simulink model "MySystem"  (Simulink 4.00)
settings: Solver=ode5  SolverMode=SingleTasking  StartTime=0.0  StopTime=999999  FixedStep=0.01  RelTol=1e-3  AbsTol=1e-6
undefined symbols (not defined in the file): ABSPositionScale, ABSPowerScale, ABSTemperatureScale, ABSVelocityScale, mex_baseaddress
libraries: simulink_extras x2
settings Model: Creator=jims  LastModifiedBy=Administrator  ExternalInput=[]  SaveTime=off  SaveOutput=off  InitialState=[]  LimitDataPoints=off  MaxDataPoints=5000  IntegerOverflowMsg=none  SimulationMode=external  RTWSystemTargetFile=rtwin.tlc  RTWOptions="-aCCOptimize=1 -aEnforceIntegerDowncast=1 -aExtMode=1 -aFoldNonRolledExpr=1 -aForceParamTrailComments=0 -aGenerateComments=1 -aGenerateReport=0 -aIncDataTypeInIds=0 -aIncHierarchyInIds=0 -aInlineInvariantSignals=0 -aInlineParameters=0 -aInlinedPrmAccess=\"Literals\" -aLocalBlockOutputs=1 -aMaxRTWIdLen=31 -aPrefixModelToSubsysFcnNames=1 -aRTWVerbose=1 -aRebuildAll=0 -aRollThreshold=5 -aShowEliminatedStatements=1"  RTWTemplateMakefile=abs_win_vc.tmf  ExtModeMexFile=rtwinext  ExtModeTrigDuration=6000  BlockReductionOpt=off

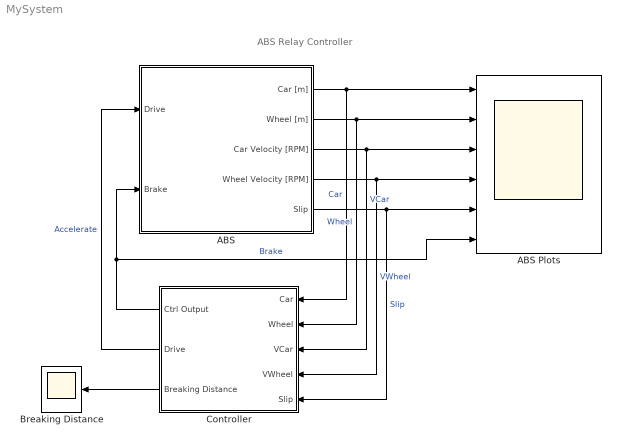
== system MySystem ==
  note: ABS Relay Controller
  ABS : Subsystem  mask{BaseAddress=mex_baseaddress(-1,-1), T0=0.01}
      mask prompts: BaseAddress "Base Address"; T0 "Sample Time"
      settings: RTWFcnNameOpts=Auto  RTWFileNameOpts=Auto
      mask Display: plot([-0.2 -0.2], [-0.2 -0.2], [1.2 1.2], [1.2 1.2], [0.9 0.9], [0.6 0.9], [0.9 0.9], [0.3 0.5], [0.85 0.85 0.95 0.95], [0.7 0.5 0.5 0.7], [0.75 0.75], [0.8 0.9], [0.75 0.75], [0.3 0.4], [0.75 0.775], [0.4 0.425], [0.775 0.725 0.775], [0.425 0.475 0.525], [0.775 0.725 0.775], [0.525 0.575 0.625], [0.775 0.725 0.775], [0.625 0.675 0.725], [0.775 0.725 0.75], [0.725 0.775 0.8], [0.65 0.95], [0.9 0.9], [0.65 0.7], [0.9 1], [0.7 0.75], [0.9 1], [0.75 0.8], [0.9 1], [0.8 0.85], [0.9 1], [0.85 0.9], [0.9 1], [0.9 0.95], [0.9 1], [0.95 1], [0.9 1], 0.4+0.3*sin([0 0.20 0.41 0.62 0.83 1.04 1.25 1.46 1.67 1.88 2.09 2.30 2.51 2.72 2.93 3.14 3.35 3.56 3.76 3.97 4.18 4.39 4.60 4.81 5.02 5.23 5.44 5.65 5.86 6.07 6.28]), 0.3+0.3*cos([0 0.20 0.41 0.62 0.83 1.04 1.25 1.46 1.67 1.88 2.09 2.30 2.51 2.72 2.93 3.14 3.35 3.56 3.76 3.97 4.18 4.39 4.60 4.81 5.02 5.23 5.44 5.65 5.86 6.07 6.28]), (1-0.005)+0.005*sin([0 0.20 0.41 0.62 0.83 1.04 1.25 1.46 1.67 1.88 2.09 2.30 2.51 2.72 2.93 3.14 3.35 3.56 3.76 3.97 4.18 4.39 4.60 4.81 5.02 5.23 5.44 5.65 5.86 6.07 6.28]), 0.3+0.005*cos([0 0.20 0.41 0.62 0.83 1.04 1.25 1.46 1.67 1.88 2.09 2.30 2.51 2.72 2.93 3.14 3.35 3.56 3.76 3.97 4.18 4.39 4.60 4.81 5.02 5.23 5.44 5.65 5.86 6.07 6.28]), 0.4+0.005*sin([0 0.20 0.41 0.62 0.83 1.04 1.25 1.46 1.67 1.88 2.09 2.30 2.51 2.72 2.93 3.14 3.35 3.56 3.76 3.97 4.18 4.39 4.60 4.81 5.02 5.23 5.44 5.65 5.86 6.07 6.28]), 0.3+0.005*cos([0 0.20 0.41 0.62 0.83 1.04 1.25 1.46 1.67 1.88 2.09 2.30 2.51 2.72 2.93 3.14 3.35 3.56 3.76 3.97 4.18 4.39 4.60 4.81 5.02 5.23 5.44 5.65 5.86 6.07 6.28]), [0.4 1], [0.3 0.3], [0 1], [0 0] )
  ABS Plots : Scope  NumInputPorts=6
      settings: TimeRange=30  YMin=0~0~0~0~-0.05~0  YMax=140~140~1750~1750~0.3~1  SaveName=ABSHistory  LimitDataPoints=on  MaxDataPoints=6000
  Breaking Distance : Scope
      settings: TimeRange=30  YMin=0  YMax=15  SaveName=ABSBreakingWay  LimitDataPoints=on  MaxDataPoints=6000
  Controller : Subsystem  Orientation=left  mask(ABS Relay Controller){VelTr=1700, SwPoint=[0.1 0.1], CntLevel=[0 1]}
      mask prompts: VelTr "Velocity Treshold [RPM]:"; SwPoint "Switch Point [ON OFF]:"; CntLevel "Control When [ON OFF]:"
      mask help: Parameters of the ABS relay controller
      settings: RTWFcnNameOpts=Auto  RTWFileNameOpts=Auto
  wires:
  Controller/2(Drive) -> ABS/1(Drive)  "Accelerate"
  Controller/1(Ctrl Output) -> ABS/2(Brake), ABS Plots/6  "Brake"
  ABS/1(Car [m]) -> Controller/1(Car), ABS Plots/1  "Car"
  ABS/2(Wheel [m]) -> Controller/2(Wheel), ABS Plots/2  "Wheel"
  ABS/3(Car Velocity [RPM]) -> Controller/3(VCar), ABS Plots/3  "VCar"
  ABS/4(Wheel Velocity [RPM]) -> Controller/4(VWheel), ABS Plots/4  "VWheel"
  ABS/5(Slip) -> Controller/5(Slip), ABS Plots/5  "Slip"
  Controller/3(Breaking Distance) -> Breaking Distance/1

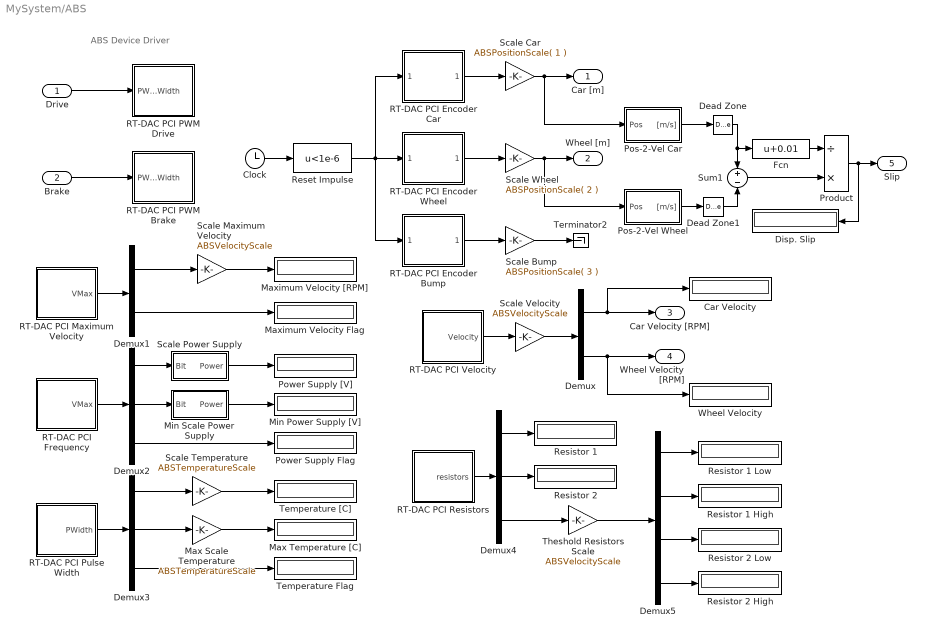
== system MySystem/ABS ==
  note: ABS Device Driver
  Drive : Inport  Port=1  LatchInput=off
  Brake : Inport  Port=2  LatchInput=off
  Car Velocity : Display
      settings: Format=short
  Clock : Clock
      settings: DisplayTime=off  Decimation=10
  Dead Zone : DeadZone  LowerValue=-0.05  UpperValue=0.05  SaturateOnIntegerOverflow=on  LinearizeAsGain=on
  Dead Zone1 : DeadZone  LowerValue=-0.05  UpperValue=0.05  SaturateOnIntegerOverflow=on  LinearizeAsGain=on
  Demux : Demux  Outputs=2  BusSelectionMode=off
  Demux1 : Demux  Outputs=2  BusSelectionMode=off
  Demux2 : Demux  Outputs=3  BusSelectionMode=off
  Demux3 : Demux  Outputs=3  BusSelectionMode=off
  Demux4 : Demux  Outputs=[1 1 4]  BusSelectionMode=off
  Demux5 : Demux  Outputs=4  BusSelectionMode=off
  Disp. Slip : Display
      settings: Format=bank
  Fcn : Fcn  Expr=u+0.01
  Max Scale Temperature : Gain  Gain=ABSTemperatureScale  Multiplication=Element-wise(K.*u)  SaturateOnIntegerOverflow=off
  Max Temperature [C] : Display
      settings: Format=short
  Maximum Velocity Flag : Display
      settings: Format=short
  Maximum Velocity [RPM] : Display
      settings: Format=short
  Min Power Supply [V] : Display
      settings: Format=short
  Min Scale Power Supply : Subsystem
      settings: RTWFcnNameOpts=Auto  RTWFileNameOpts=Auto
  Pos-2-Vel Car : Subsystem
      settings: RTWFcnNameOpts=Auto  RTWFileNameOpts=Auto
  Pos-2-Vel Wheel : Subsystem
      settings: RTWFcnNameOpts=Auto  RTWFileNameOpts=Auto
  Power Supply Flag : Display
      settings: Format=short
  Power Supply [V] : Display
      settings: Format=short
  Product : Product  Inputs=/*  Multiplication=Element-wise(.*)  SaturateOnIntegerOverflow=on
  RT-DAC PCI Encoder Bump : Subsystem  mask(Incremental Encoders){BaseAddress=BaseAddress, ChannelIdx=2, T0=T0}
      mask prompts: BaseAddress "Base Address:"; ChannelIdx "Channel:"; T0 "Sample Time (sec):"
      mask help: RT-DAC PCI Device Driver
      settings: RTWFcnNameOpts=Auto  RTWFileNameOpts=Auto
      mask Help: Set up each field for your specific hardware configuration.
      mask StyleString: edit,popup(0|1|2|3),edit
      mask Display: plot(0,0,100,100,[90,80,80,11,11],[90,90,20,20,80],[11,80],[80,80],[80,80],[20,14],[80,85,85,80],[45,45,66,66],[45,45,74,74],[20,13,13,20],[15,27,27,15,15],[75,75,26,26,75],[33,48,48,33,33],[75,75,55,55,75],[55,55,71,71,55],[55,75,75,55,55],[33,41,41,33,33],[50,50,27,27,50],[48,56,56,48,48],[50,50,27,27,50],[62,70,70,62,62],[50,50,27,27,50])
  RT-DAC PCI Encoder Car : Subsystem  mask(Incremental Encoders){BaseAddress=BaseAddress, ChannelIdx=0, T0=T0}
      mask prompts: BaseAddress "Base Address:"; ChannelIdx "Channel:"; T0 "Sample Time (sec):"
      mask help: RT-DAC PCI Device Driver
      settings: RTWFcnNameOpts=Auto  RTWFileNameOpts=Auto
      mask Help: Set up each field for your specific hardware configuration.
      mask StyleString: edit,popup(0|1|2|3),edit
      mask Display: plot(0,0,100,100,[90,80,80,11,11],[90,90,20,20,80],[11,80],[80,80],[80,80],[20,14],[80,85,85,80],[45,45,66,66],[45,45,74,74],[20,13,13,20],[15,27,27,15,15],[75,75,26,26,75],[33,48,48,33,33],[75,75,55,55,75],[55,55,71,71,55],[55,75,75,55,55],[33,41,41,33,33],[50,50,27,27,50],[48,56,56,48,48],[50,50,27,27,50],[62,70,70,62,62],[50,50,27,27,50])
  RT-DAC PCI Encoder Wheel : Subsystem  mask(Incremental Encoders){BaseAddress=BaseAddress, ChannelIdx=1, T0=T0}
      mask prompts: BaseAddress "Base Address:"; ChannelIdx "Channel:"; T0 "Sample Time (sec):"
      mask help: RT-DAC PCI Device Driver
      settings: RTWFcnNameOpts=Auto  RTWFileNameOpts=Auto
      mask Help: Set up each field for your specific hardware configuration.
      mask StyleString: edit,popup(0|1|2|3),edit
      mask Display: plot(0,0,100,100,[90,80,80,11,11],[90,90,20,20,80],[11,80],[80,80],[80,80],[20,14],[80,85,85,80],[45,45,66,66],[45,45,74,74],[20,13,13,20],[15,27,27,15,15],[75,75,26,26,75],[33,48,48,33,33],[75,75,55,55,75],[55,55,71,71,55],[55,75,75,55,55],[33,41,41,33,33],[50,50,27,27,50],[48,56,56,48,48],[50,50,27,27,50],[62,70,70,62,62],[50,50,27,27,50])
  RT-DAC PCI Frequency : Subsystem  mask(Incremental Encoders){BaseAddress=BaseAddress, T0=T0}
      mask prompts: BaseAddress "Base Address:"; T0 "Sample Time (sec):"
      mask help: RT-DAC PCI Device Driver
      settings: RTWFcnNameOpts=Auto  RTWFileNameOpts=Auto
      mask Help: Set up each field for your specific hardware configuration.
      mask Display: plot(0,0,100,100,[90,80,80,11,11],[90,90,20,20,80],[11,80],[80,80],[80,80],[20,14],[80,85,85,80],[45,45,66,66],[45,45,74,74],[20,13,13,20],[15,27,27,15,15],[75,75,26,26,75],[33,48,48,33,33],[75,75,55,55,75],[55,55,71,71,55],[55,75,75,55,55],[33,41,41,33,33],[50,50,27,27,50],[48,56,56,48,48],[50,50,27,27,50],[62,70,70,62,62],[50,50,27,27,50])
  RT-DAC PCI Maximum Velocity : Subsystem  mask(Incremental Encoders){BaseAddress=BaseAddress, T0=T0}
      mask prompts: BaseAddress "Base Address:"; T0 "Sample Time (sec):"
      mask help: RT-DAC PCI Device Driver
      settings: RTWFcnNameOpts=Auto  RTWFileNameOpts=Auto
      mask Help: Set up each field for your specific hardware configuration.
      mask Display: plot(0,0,100,100,[90,80,80,11,11],[90,90,20,20,80],[11,80],[80,80],[80,80],[20,14],[80,85,85,80],[45,45,66,66],[45,45,74,74],[20,13,13,20],[15,27,27,15,15],[75,75,26,26,75],[33,48,48,33,33],[75,75,55,55,75],[55,55,71,71,55],[55,75,75,55,55],[33,41,41,33,33],[50,50,27,27,50],[48,56,56,48,48],[50,50,27,27,50],[62,70,70,62,62],[50,50,27,27,50])
  RT-DAC PCI PWM Brake : Subsystem  mask(PWM Module){BaseAddress=BaseAddress, ChanIdx=1, ChanMode=12 Bit, ChanPresc=60, SetOutputsFlag=on, SetOutputsValue=0, T0=T0}
      mask prompts: BaseAddress "IO Base Address:"; ChanIdx "Channel:"; ChanMode "Channel Mode:"; ChanPresc "Channel Prescaler:"; SetOutputsFlag "Set Outputs At Termination"; SetOutputsValue "Termination Outputs:"; T0 "Sample Time (sec):"
      mask help: RT-DAC PCI Device Driver
      settings: RTWFcnNameOpts=Auto  RTWFileNameOpts=Auto
      mask Help: Set up each field for your specific hardware configuration.
      mask StyleString: edit,popup(0|1|2|3),popup(8 Bit|12 Bit),edit,checkbox,edit,edit
      mask Display: plot(0,0,100,100,[90,80,80,11,11],[90,90,20,20,80],[11,80],[80,80],[80,80],[20,14],[80,85,85,80],[45,45,66,66],[45,45,74,74],[20,13,13,20],[15,27,27,15,15],[75,75,26,26,75],[33,48,48,33,33],[75,75,55,55,75],[55,55,71,71,55],[55,75,75,55,55],[33,41,41,33,33],[50,50,27,27,50],[48,56,56,48,48],[50,50,27,27,50],[62,70,70,62,62],[50,50,27,27,50])
  RT-DAC PCI PWM Drive : Subsystem  mask(PWM Module){BaseAddress=BaseAddress, ChanIdx=0, ChanMode=12 Bit, ChanPresc=60, SetOutputsFlag=on, SetOutputsValue=0, T0=T0}
      mask prompts: BaseAddress "IO Base Address:"; ChanIdx "Channel:"; ChanMode "Channel Mode:"; ChanPresc "Channel Prescaler:"; SetOutputsFlag "Set Outputs At Termination"; SetOutputsValue "Termination Outputs:"; T0 "Sample Time (sec):"
      mask help: RT-DAC PCI Device Driver
      settings: RTWFcnNameOpts=Auto  RTWFileNameOpts=Auto
      mask Help: Set up each field for your specific hardware configuration.
      mask StyleString: edit,popup(0|1|2|3),popup(8 Bit|12 Bit),edit,checkbox,edit,edit
      mask Display: plot(0,0,100,100,[90,80,80,11,11],[90,90,20,20,80],[11,80],[80,80],[80,80],[20,14],[80,85,85,80],[45,45,66,66],[45,45,74,74],[20,13,13,20],[15,27,27,15,15],[75,75,26,26,75],[33,48,48,33,33],[75,75,55,55,75],[55,55,71,71,55],[55,75,75,55,55],[33,41,41,33,33],[50,50,27,27,50],[48,56,56,48,48],[50,50,27,27,50],[62,70,70,62,62],[50,50,27,27,50])
  RT-DAC PCI Pulse Width : Subsystem  mask(Incremental Encoders){BaseAddress=BaseAddress, T0=T0}
      mask prompts: BaseAddress "Base Address:"; T0 "Sample Time (sec):"
      mask help: RT-DAC PCI Device Driver
      settings: RTWFcnNameOpts=Auto  RTWFileNameOpts=Auto
      mask Help: Set up each field for your specific hardware configuration.
      mask Display: plot(0,0,100,100,[90,80,80,11,11],[90,90,20,20,80],[11,80],[80,80],[80,80],[20,14],[80,85,85,80],[45,45,66,66],[45,45,74,74],[20,13,13,20],[15,27,27,15,15],[75,75,26,26,75],[33,48,48,33,33],[75,75,55,55,75],[55,55,71,71,55],[55,75,75,55,55],[33,41,41,33,33],[50,50,27,27,50],[48,56,56,48,48],[50,50,27,27,50],[62,70,70,62,62],[50,50,27,27,50])
  RT-DAC PCI Resistors : Subsystem  mask(Incremental Encoders){BaseAddress=BaseAddress, T0=T0}
      mask prompts: BaseAddress "Base Address:"; T0 "Sample Time (sec):"
      mask help: RT-DAC PCI Device Driver
      settings: RTWFcnNameOpts=Auto  RTWFileNameOpts=Auto
      mask Help: Set up each field for your specific hardware configuration.
      mask Display: plot(0,0,100,100,[90,80,80,11,11],[90,90,20,20,80],[11,80],[80,80],[80,80],[20,14],[80,85,85,80],[45,45,66,66],[45,45,74,74],[20,13,13,20],[15,27,27,15,15],[75,75,26,26,75],[33,48,48,33,33],[75,75,55,55,75],[55,55,71,71,55],[55,75,75,55,55],[33,41,41,33,33],[50,50,27,27,50],[48,56,56,48,48],[50,50,27,27,50],[62,70,70,62,62],[50,50,27,27,50])
  RT-DAC PCI Velocity : Subsystem  mask(Incremental Encoders){BaseAddress=BaseAddress, T0=T0}
      mask prompts: BaseAddress "Base Address:"; T0 "Sample Time (sec):"
      mask help: RT-DAC PCI Device Driver
      settings: RTWFcnNameOpts=Auto  RTWFileNameOpts=Auto
      mask Help: Set up each field for your specific hardware configuration.
      mask Display: plot(0,0,100,100,[90,80,80,11,11],[90,90,20,20,80],[11,80],[80,80],[80,80],[20,14],[80,85,85,80],[45,45,66,66],[45,45,74,74],[20,13,13,20],[15,27,27,15,15],[75,75,26,26,75],[33,48,48,33,33],[75,75,55,55,75],[55,55,71,71,55],[55,75,75,55,55],[33,41,41,33,33],[50,50,27,27,50],[48,56,56,48,48],[50,50,27,27,50],[62,70,70,62,62],[50,50,27,27,50])
  Reset Impulse : Fcn  Expr=u<1e-6
  Resistor 1 : Display
      settings: Format=short
  Resistor 1 High : Display
      settings: Format=short
  Resistor 1 Low : Display
      settings: Format=short
  Resistor 2 : Display
      settings: Format=short
  Resistor 2 High : Display
      settings: Format=short
  Resistor 2 Low : Display
      settings: Format=short
  Scale Bump : Gain  Gain=ABSPositionScale( 3 )  Multiplication=Element-wise(K.*u)  SaturateOnIntegerOverflow=off
  Scale Car : Gain  Gain=ABSPositionScale( 1 )  Multiplication=Element-wise(K.*u)  SaturateOnIntegerOverflow=off
  Scale Maximum Velocity : Gain  Gain=ABSVelocityScale  Multiplication=Element-wise(K.*u)  SaturateOnIntegerOverflow=off
  Scale Velocity : Gain  Gain=ABSVelocityScale  Multiplication=Element-wise(K.*u)  SaturateOnIntegerOverflow=off
  Scale Wheel : Gain  Gain=ABSPositionScale( 2 )  Multiplication=Element-wise(K.*u)  SaturateOnIntegerOverflow=off
  Scale Power Supply : Subsystem
      settings: RTWFcnNameOpts=Auto  RTWFileNameOpts=Auto
  Scale Temperature : Gain  Gain=ABSTemperatureScale  Multiplication=Element-wise(K.*u)  SaturateOnIntegerOverflow=off
  Sum1 : Sum  Inputs=+-  SaturateOnIntegerOverflow=on
  Temperature Flag : Display
      settings: Format=short
  Temperature [C] : Display
      settings: Format=short
  Terminator2 : Terminator
  Theshold Resistors Scale : Gain  Gain=ABSVelocityScale  Multiplication=Element-wise(K.*u)  SaturateOnIntegerOverflow=off
  Wheel Velocity : Display
      settings: Format=short
  Car [m] : Outport  Port=1
  Wheel [m] : Outport  Port=2
  Car Velocity [RPM] : Outport  Port=3
  Wheel Velocity [RPM] : Outport  Port=4
  Slip : Outport  Port=5
  wires:
  Dead Zone1/1 -> Sum1/2
  Dead Zone/1 -> Fcn/1, Sum1/1
  Pos-2-Vel Car/1("[m/s]") -> Dead Zone/1
  Pos-2-Vel Wheel/1("[m/s]") -> Dead Zone1/1
  Product/1 -> Disp. Slip/1, Slip/1
  Fcn/1 -> Product/1
  Sum1/1 -> Product/2
  Demux5/4 -> Resistor 2 High/1
  Demux5/3 -> Resistor 2 Low/1
  Demux5/2 -> Resistor 1 High/1
  Demux5/1 -> Resistor 1 Low/1
  Theshold Resistors Scale/1 -> Demux5/1
  Demux4/3 -> Theshold Resistors Scale/1
  Demux4/2 -> Resistor 2/1
  Demux4/1 -> Resistor 1/1
  RT-DAC PCI Resistors/1(resistors) -> Demux4/1
  Demux3/3 -> Temperature Flag/1
  Demux3/2 -> Max Scale Temperature/1
  Max Scale Temperature/1 -> Max Temperature [C]/1
  Demux2/3 -> Power Supply Flag/1
  Min Scale Power Supply/1(Power) -> Min Power Supply [V]/1
  Demux2/2 -> Min Scale Power Supply/1(Bit)
  Reset Impulse/1 -> RT-DAC PCI Encoder Bump/1(Reset), RT-DAC PCI Encoder Car/1(Reset), RT-DAC PCI Encoder Wheel/1(Reset)
  Clock/1 -> Reset Impulse/1
  Demux3/1 -> Scale Temperature/1
  RT-DAC PCI Pulse Width/1(PWidth) -> Demux3/1
  Demux2/1 -> Scale Power Supply/1(Bit)
  RT-DAC PCI Frequency/1(VMax) -> Demux2/1
  Demux1/2 -> Maximum Velocity Flag/1
  Scale Maximum Velocity/1 -> Maximum Velocity [RPM]/1
  Demux1/1 -> Scale Maximum Velocity/1
  RT-DAC PCI Maximum Velocity/1(VMax) -> Demux1/1
  Demux/2 -> Wheel Velocity/1, Wheel Velocity [RPM]/1
  Demux/1 -> Car Velocity/1, Car Velocity [RPM]/1
  Brake/1 -> RT-DAC PCI PWM Brake/1(PWM Width)
  Drive/1 -> RT-DAC PCI PWM Drive/1(PWM Width)
  Scale Temperature/1 -> Temperature [C]/1
  Scale Power Supply/1(Power) -> Power Supply [V]/1
  Scale Velocity/1 -> Demux/1
  RT-DAC PCI Velocity/1(Velocity) -> Scale Velocity/1
  Scale Bump/1 -> Terminator2/1
  Scale Wheel/1 -> Pos-2-Vel Wheel/1(Pos), Wheel [m]/1
  Scale Car/1 -> Pos-2-Vel Car/1(Pos), Car [m]/1
  RT-DAC PCI Encoder Bump/1(Encoder Counter) -> Scale Bump/1
  RT-DAC PCI Encoder Wheel/1(Encoder Counter) -> Scale Wheel/1
  RT-DAC PCI Encoder Car/1(Encoder Counter) -> Scale Car/1

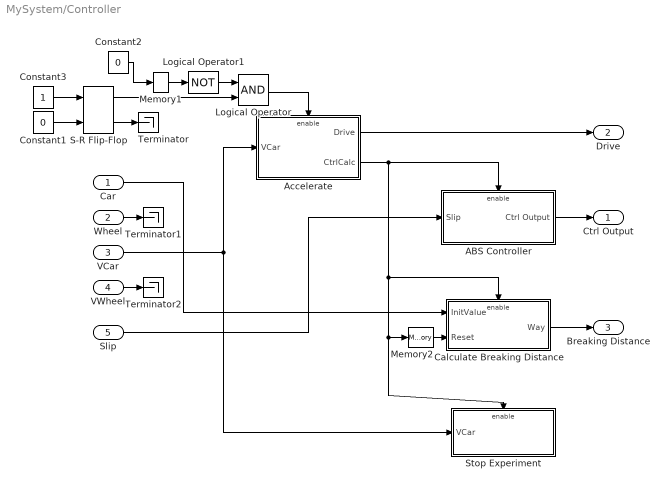
== system MySystem/Controller ==
  Car : Inport  Port=1  LatchInput=off
  Wheel : Inport  Port=2  LatchInput=off
  VCar : Inport  Port=3  LatchInput=off
  VWheel : Inport  Port=4  LatchInput=off
  Slip : Inport  Port=5  LatchInput=off
  ABS Controller : Subsystem  TreatAsAtomicUnit=on
      settings: RTWFcnNameOpts=Auto  RTWFileNameOpts=Auto
  Accelerate : Subsystem  TreatAsAtomicUnit=on
      settings: RTWFcnNameOpts=Auto  RTWFileNameOpts=Auto
  Calculate Breaking Distance : Subsystem  TreatAsAtomicUnit=on
      settings: RTWFcnNameOpts=Auto  RTWFileNameOpts=Auto
  Constant1 : Constant  Value=0
  Constant2 : Constant  Value=0
  Constant3 : Constant  Value=1
  Logical Operator : Logic  Operator=AND  Inputs=2
  Logical Operator1 : Logic  Operator=NOT  Inputs=2
  Memory1 : Memory  X0=0  InheritSampleTime=off
      settings: RTWStateStorageClass=Auto
  Memory2 : Memory  X0=0  InheritSampleTime=off
      settings: RTWStateStorageClass=Auto
  S-R Flip-Flop : simulink_extras/Flip Flops/S-R Flip-Flop  initial_condition=0
  Stop Experiment : Subsystem  TreatAsAtomicUnit=on
      settings: RTWFcnNameOpts=Auto  RTWFileNameOpts=Auto
  Terminator : Terminator
  Terminator1 : Terminator
  Terminator2 : Terminator
  Ctrl Output : Outport  Port=1
  Drive : Outport  Port=2
  Breaking Distance : Outport  Port=3
  wires:
  Logical Operator1/1 -> Logical Operator/1
  S-R Flip-Flop/1 -> Logical Operator/2
  Logical Operator/1 -> Accelerate/Enable
  Accelerate/2(CtrlCalc) -> ABS Controller/Enable, Calculate Breaking Distance/Enable, Memory2/1, Stop Experiment/Enable
  S-R Flip-Flop/2 -> Terminator/1
  Constant1/1 -> S-R Flip-Flop/2
  Accelerate/1(Drive) -> Drive/1
  ABS Controller/1(Ctrl Output) -> Ctrl Output/1
  Calculate Breaking Distance/1(Way) -> Breaking Distance/1
  VCar/1 -> Accelerate/1(VCar), Stop Experiment/1(VCar)
  Car/1 -> Calculate Breaking Distance/1(InitValue)
  Memory2/1 -> Calculate Breaking Distance/2(Reset)
  Memory1/1 -> Logical Operator1/1
  Slip/1 -> ABS Controller/1(Slip)
  Constant2/1 -> Memory1/1
  Constant3/1 -> S-R Flip-Flop/1
  Wheel/1 -> Terminator1/1
  VWheel/1 -> Terminator2/1

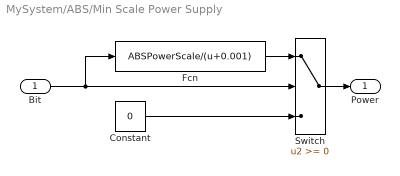
== system MySystem/ABS/Min Scale Power Supply ==
  Bit : Inport  Port=1  LatchInput=off
  Constant : Constant  Value=0
  Fcn : Fcn  Expr=ABSPowerScale/(u+0.001)
  Switch : Switch  Threshold=0
  Power : Outport  Port=1
  wires:
  Bit/1 -> Switch/2, Fcn/1
  Switch/1 -> Power/1
  Fcn/1 -> Switch/1
  Constant/1 -> Switch/3

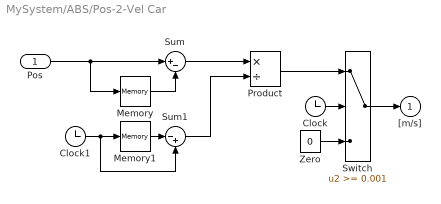
== system MySystem/ABS/Pos-2-Vel Car ==
  Pos : Inport  Port=1  LatchInput=off
  Clock : Clock
      settings: DisplayTime=off  Decimation=10
  Clock1 : Clock
      settings: DisplayTime=off  Decimation=10
  Memory : Memory  X0=0  InheritSampleTime=on
      settings: RTWStateStorageClass=Auto
  Memory1 : Memory  X0=0  InheritSampleTime=on
      settings: RTWStateStorageClass=Auto
  Product : Product  Inputs=*/  Multiplication=Element-wise(.*)  SaturateOnIntegerOverflow=on
  Sum : Sum  Inputs=|+-  SaturateOnIntegerOverflow=on
  Sum1 : Sum  Inputs=|-+  SaturateOnIntegerOverflow=on
  Switch : Switch  Threshold=0.001
  Zero : Constant  Value=0
  "[m/s]" : Outport  Port=1  InitialOutput=0
  wires:
  Pos/1 -> Memory/1, Sum/1
  Memory/1 -> Sum/2
  Clock/1 -> Switch/2
  Switch/1 -> "[m/s]"/1
  Zero/1 -> Switch/3
  Product/1 -> Switch/1
  Sum/1 -> Product/1
  Clock1/1 -> Memory1/1, Sum1/2
  Memory1/1 -> Sum1/1
  Sum1/1 -> Product/2

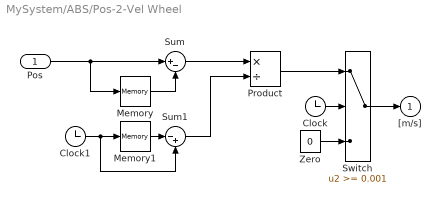
== system MySystem/ABS/Pos-2-Vel Wheel ==
  Pos : Inport  Port=1  LatchInput=off
  Clock : Clock
      settings: DisplayTime=off  Decimation=10
  Clock1 : Clock
      settings: DisplayTime=off  Decimation=10
  Memory : Memory  X0=0  InheritSampleTime=on
      settings: RTWStateStorageClass=Auto
  Memory1 : Memory  X0=0  InheritSampleTime=on
      settings: RTWStateStorageClass=Auto
  Product : Product  Inputs=*/  Multiplication=Element-wise(.*)  SaturateOnIntegerOverflow=on
  Sum : Sum  Inputs=|+-  SaturateOnIntegerOverflow=on
  Sum1 : Sum  Inputs=|-+  SaturateOnIntegerOverflow=on
  Switch : Switch  Threshold=0.001
  Zero : Constant  Value=0
  "[m/s]" : Outport  Port=1  InitialOutput=0
  wires:
  Sum1/1 -> Product/2
  Memory1/1 -> Sum1/1
  Clock1/1 -> Sum1/2, Memory1/1
  Sum/1 -> Product/1
  Product/1 -> Switch/1
  Zero/1 -> Switch/3
  Switch/1 -> "[m/s]"/1
  Clock/1 -> Switch/2
  Memory/1 -> Sum/2
  Pos/1 -> Sum/1, Memory/1

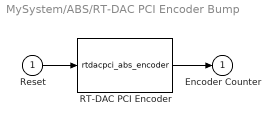
== system MySystem/ABS/RT-DAC PCI Encoder Bump ==
  Reset : Inport  Port=1  LatchInput=off
  RT-DAC PCI Encoder : S-Function  FunctionName=rtdacpci_abs_encoder  Parameters=BaseAddress, ChannelIdx, T0  PortCounts=[]  SFunctionModules=''
  Encoder Counter : Outport  Port=1  InitialOutput=0
  wires:
  RT-DAC PCI Encoder/1 -> Encoder Counter/1
  Reset/1 -> RT-DAC PCI Encoder/1

== system MySystem/ABS/RT-DAC PCI Encoder Car ==
  Reset : Inport  Port=1  LatchInput=off
  RT-DAC PCI Encoder : S-Function  FunctionName=rtdacpci_abs_encoder  Parameters=BaseAddress, ChannelIdx, T0  PortCounts=[]  SFunctionModules=''
  Encoder Counter : Outport  Port=1  InitialOutput=0
  wires:
  RT-DAC PCI Encoder/1 -> Encoder Counter/1
  Reset/1 -> RT-DAC PCI Encoder/1

== system MySystem/ABS/RT-DAC PCI Encoder Wheel ==
  Reset : Inport  Port=1  LatchInput=off
  RT-DAC PCI Encoder : S-Function  FunctionName=rtdacpci_abs_encoder  Parameters=BaseAddress, ChannelIdx, T0  PortCounts=[]  SFunctionModules=''
  Encoder Counter : Outport  Port=1  InitialOutput=0
  wires:
  Reset/1 -> RT-DAC PCI Encoder/1
  RT-DAC PCI Encoder/1 -> Encoder Counter/1

== system MySystem/ABS/RT-DAC PCI Frequency ==
  RT-DAC PCI Frequency : S-Function  FunctionName=rtdacpci_abs_frequency  Parameters=BaseAddress, T0  PortCounts=[]  SFunctionModules=''
  VMax : Outport  Port=1  InitialOutput=0
  wires:
  RT-DAC PCI Frequency/1 -> VMax/1

== system MySystem/ABS/RT-DAC PCI Maximum Velocity ==
  RT-DAC PCI VMax : S-Function  FunctionName=rtdacpci_abs_vmax  Parameters=BaseAddress, T0  PortCounts=[]  SFunctionModules=''
  VMax : Outport  Port=1  InitialOutput=0
  wires:
  RT-DAC PCI VMax/1 -> VMax/1

== system MySystem/ABS/RT-DAC PCI PWM Brake ==
  PWM Width : Inport  Port=1  LatchInput=off
  "RT-DAC PCI PWM " : S-Function  FunctionName=rtdacpci_abs_pwm  Parameters=BaseAddress, ChanIdx, ChanMode, ChanPresc, SetOutputsFlag, SetOutputsValue, T0  PortCounts=[]  SFunctionModules=''
  wires:
  PWM Width/1 -> "RT-DAC PCI PWM "/1

== system MySystem/ABS/RT-DAC PCI PWM Drive ==
  PWM Width : Inport  Port=1  LatchInput=off
  "RT-DAC PCI PWM " : S-Function  FunctionName=rtdacpci_abs_pwm  Parameters=BaseAddress, ChanIdx, ChanMode, ChanPresc, SetOutputsFlag, SetOutputsValue, T0  PortCounts=[]  SFunctionModules=''
  wires:
  PWM Width/1 -> "RT-DAC PCI PWM "/1

== system MySystem/ABS/RT-DAC PCI Pulse Width ==
  RT-DAC PCI Pulse Width : S-Function  FunctionName=rtdacpci_abs_pulsewidth  Parameters=BaseAddress, T0  PortCounts=[]  SFunctionModules=''
  PWidth : Outport  Port=1  InitialOutput=0
  wires:
  RT-DAC PCI Pulse Width/1 -> PWidth/1

== system MySystem/ABS/RT-DAC PCI Resistors ==
  RT-DAC PCI Resistors : S-Function  FunctionName=rtdacpci_abs_resistors  Parameters=BaseAddress, T0  PortCounts=[]  SFunctionModules=''
  resistors : Outport  Port=1  InitialOutput=0
  wires:
  RT-DAC PCI Resistors/1 -> resistors/1

== system MySystem/ABS/RT-DAC PCI Velocity ==
  RT-DAC PCI Velocity : S-Function  FunctionName=rtdacpci_abs_velocity  Parameters=BaseAddress, T0  PortCounts=[]  SFunctionModules=''
  Velocity : Outport  Port=1  InitialOutput=0
  wires:
  RT-DAC PCI Velocity/1 -> Velocity/1

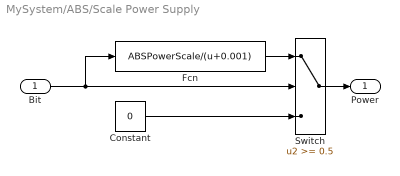
== system MySystem/ABS/Scale Power Supply ==
  Bit : Inport  Port=1  LatchInput=off
  Constant : Constant  Value=0
  Fcn : Fcn  Expr=ABSPowerScale/(u+0.001)
  Switch : Switch  Threshold=0.5
  Power : Outport  Port=1
  wires:
  Constant/1 -> Switch/3
  Fcn/1 -> Switch/1
  Switch/1 -> Power/1
  Bit/1 -> Fcn/1, Switch/2

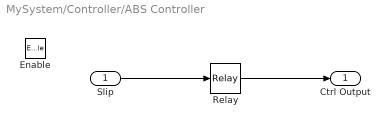
== system MySystem/Controller/ABS Controller ==
  Slip : Inport  Port=1  LatchInput=off
  Enable : EnablePort
  Relay : Relay  OnSwitchValue=SwPoint(1)  OffSwitchValue=SwPoint(2)  OnOutputValue=CntLevel(1)  OffOutputValue=CntLevel(2)
  Ctrl Output : Outport  Port=1
  wires:
  Slip/1 -> Relay/1
  Relay/1 -> Ctrl Output/1

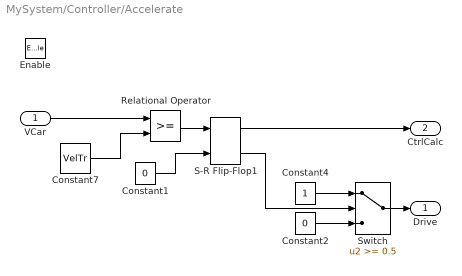
== system MySystem/Controller/Accelerate ==
  VCar : Inport  Port=1  LatchInput=off
  Enable : EnablePort
  Constant1 : Constant  Value=0
  Constant2 : Constant  Value=0
  Constant4 : Constant  Value=1
  Constant7 : Constant  Value=VelTr
  Relational Operator : RelationalOperator  Operator=>=
  S-R Flip-Flop1 : simulink_extras/Flip Flops/S-R Flip-Flop  initial_condition=0
  Switch : Switch  Threshold=0.5
  Drive : Outport  Port=1
  CtrlCalc : Outport  Port=2
  wires:
  Constant7/1 -> Relational Operator/2
  Relational Operator/1 -> S-R Flip-Flop1/1
  VCar/1 -> Relational Operator/1
  Constant1/1 -> S-R Flip-Flop1/2
  Switch/1 -> Drive/1
  S-R Flip-Flop1/2 -> Switch/2
  Constant2/1 -> Switch/3
  S-R Flip-Flop1/1 -> CtrlCalc/1
  Constant4/1 -> Switch/1

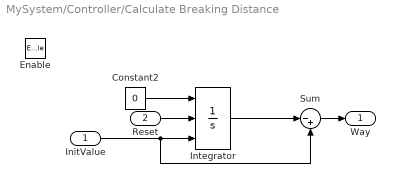
== system MySystem/Controller/Calculate Breaking Distance ==
  InitValue : Inport  Port=1  LatchInput=off
  Reset : Inport  Port=2  LatchInput=off
  Enable : EnablePort
  Constant2 : Constant  Value=0
  Integrator : Integrator  ExternalReset=rising  InitialConditionSource=external  InitialCondition=0  LimitOutput=off  UpperSaturationLimit=inf  LowerSaturationLimit=-inf  ShowSaturationPort=off  ShowStatePort=off  AbsoluteTolerance=auto
  Sum : Sum  Inputs=|-+  SaturateOnIntegerOverflow=on
  Way : Outport  Port=1
  wires:
  Constant2/1 -> Integrator/1
  Integrator/1 -> Sum/1
  InitValue/1 -> Sum/2, Integrator/3
  Reset/1 -> Integrator/2
  Sum/1 -> Way/1

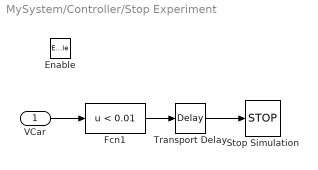
== system MySystem/Controller/Stop Experiment ==
  VCar : Inport  Port=1  LatchInput=off
  Enable : EnablePort
  Fcn1 : Fcn  Expr=u < 0.01
  Stop Simulation : Stop
  Transport Delay : TransportDelay  DelayTime=0.5  InitialInput=0  BufferSize=1024  PadeOrder=0
  wires:
  Fcn1/1 -> Transport Delay/1
  Transport Delay/1 -> Stop Simulation/1
  VCar/1 -> Fcn1/1
